simulink model "WindPlatform"  (Simulink 7.5)
settings: Solver=ode23s  StartTime=0.0  StopTime=700  RelTol=1e-3
InitFcn:
  | initialise
values from neighbouring files (symbols this model uses):
  B = 20/100    (= 0.2)    [initialise.m]    (also in windmodel.m)
  D = [6.5541e-04 0 0;0 7.1768e-04 -6.3413E-08;0 -2.1033E-08 -2.6495E-10]    [initialise.m]
  L = 30/100    (= 0.3)    [initialise.m]    (also in windmodel.m = 0.2)
  MA = [2.5 0 0 ... (first row only)    [initialise.m]
  MRB = [1.65 0 0 ... (first row only)    [initialise.m]
undefined symbols (not defined in the file or in its folder): effoceancurrent, magnitude, rotation, windmodel
libraries: simulink x3, marine_gnc x2, simulink_extras x2, instrumentlib x1, dspmtrx3 x1, aerolibutil x1
settings Model: Creator=Prasad  LastModifiedBy=Prasad
settings DebuggingCC: SolverPrmCheckMsg=none
settings SimEventsCC: propDiagAttribOutput=1  propDiagFcnCallOutput=1  propDiagStatOutput=0

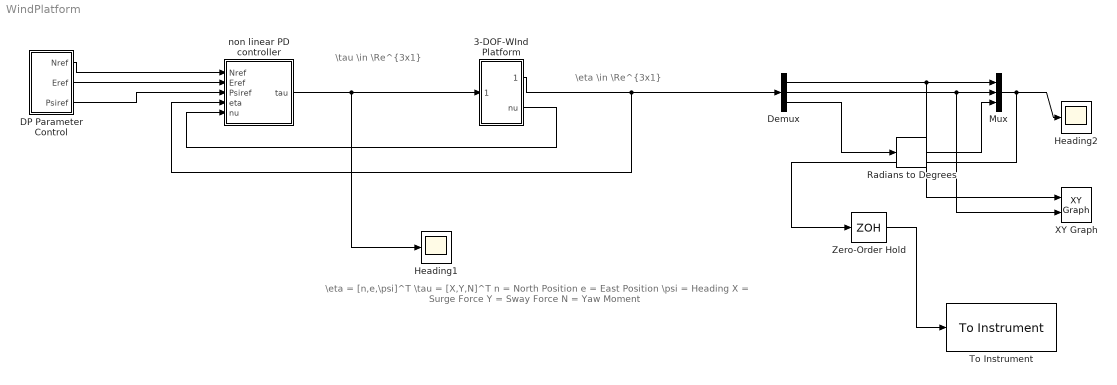
== system WindPlatform ==
  note: \tau \in \Re^{3x1}
  note: \eta \in \Re^{3x1}
  note: \eta = [n,e,\psi]^T
      | \tau = [X,Y,N]^T
      | n = North Position
      | e = East Position
      | \psi = Heading
      | X = Surge Force
      | Y = Sway Force
      | N = Yaw Moment
  3-DOF-WInd Platform : Subsystem
  DP Parameter Control : Subsystem  mask(Dynamic Position   ){geo=[10,20,100], k=[1 1 1], w=[0.05 0.05 0.05], zeta=[0.8 0.8 0.6]}
      mask prompts: geo "North-East-Heading[n,e,psi]"; k "Gain: [North East Heading]"; w "Time Constant: [North East Heading]"; zeta "Damping Factor: [North East Heading]"
      mask help: Set North-East(n,e) Positions of the vessel relative to the local geographical frame along with the heading angle relative to the north
      mask TabNameString: Basic,Advance,Advance,Advance
  Demux : Demux  Outputs=3
  Heading1 : Scope
      settings: TimeRange=700  YMin=-0.1  YMax=0.09
  Heading2 : Scope
      settings: TimeRange=700  YMin=-1  YMax=13
  Mux : Mux  Inputs=3
  Radians to Degrees : simulink_extras/Transformations/Radians to Degrees  SystemSampleTime=-1
  To Instrument : instrumentlib/To Instrument  sampleTime=-1  isWorkspaceObject=off  timeout=10  inputBufferSize=8192  protocol=UDP  serialPort=COM4  baudRate=9600  gpibVendor=Advantech  boardIndex=0  primaryAddress=1  secondaryAddress=0  visaVendor=Agilent  visaSerialPort=0  chassisIndex=0  logicalAddress=0  tcpRemoteHost='127.0.0.1'  tcpRemotePort=4500  udpRemoteHost='127.0.0.1'  udpRemotePort=9090  visaTCPBoardIndex=0  visaTCPRemoteHost='127.0.0.1'  usbBoardIndex=0  usbManufID=0  usbModelCode=0  usbSerialNumber=0  initAction=None  initCommand='DATA:SOURCE CH1'  initFunction=get  command='uw'  sendFormat=ASCII  asciiFormatting='%d'  precision=8-bit integer  byteOrder=Little endian
  XY Graph : simulink/Sinks/XY Graph  SystemSampleTime=-1  xmin=0  xmax=50  ymin=0  ymax=50  st=-1
  Zero-Order Hold : ZeroOrderHold
  non linear PD controller : Subsystem  mask(Non-Linear PD controller){kp=50*[1 0 0;1 0 0;0 0 2], kd=50}
      mask prompts: kp "Proportional Gain Kp"; kd "Derivative Gain Kd"
      mask help: Set proportional and derivative gains for the non-linear PD controller
  wires:
  Demux/1 -> Mux/1, XY Graph/1
  Demux/2 -> Mux/2, XY Graph/2
  Radians to Degrees/1 -> Mux/3
  DP Parameter Control/2(Eref) -> non linear PD controller/2(Eref)
  DP Parameter Control/1(Nref) -> non linear PD controller/1(Nref)
  Demux/3 -> Radians to Degrees/1
  3-DOF-WInd Platform/1(eta) -> non linear PD controller/4(eta), Demux/1
  3-DOF-WInd Platform/2(nu) -> non linear PD controller/5(nu)
  DP Parameter Control/3(Psiref) -> non linear PD controller/3(Psiref)
  non linear PD controller/1(tau) -> 3-DOF-WInd Platform/1(tau), Heading1/1
  Mux/1 -> Heading2/1, Zero-Order Hold/1
  Zero-Order Hold/1 -> To Instrument/1

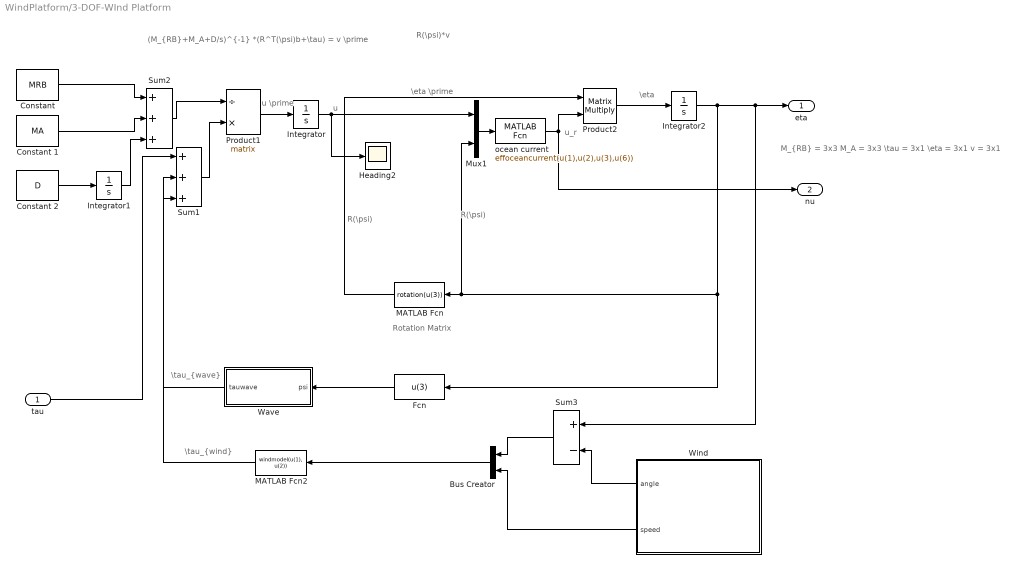
== system WindPlatform/3-DOF-WInd Platform ==
  note: (M_{RB}+M_A+D/s)^{-1} *(R^T(\psi)b+\tau) = v \prime
  note: \nu
  note: R(\psi)*v
  note: \eta
  note: M_{RB} = 3x3
      | M_A = 3x3
      | \tau = 3x1
      | \eta = 3x1
      | v = 3x1
  note: \nu \prime
  note: \eta \prime
  note: \tau_{wind}
  note: \nu_r
  note: \tau_{wave}
  note: R(\psi)
  note: R(\psi)
  note: Rotation Matrix
  tau : Inport  OutDataType=sfix(16)  OutScaling=2^0
  Bus Creator : BusCreator  Inputs=2
  "Constant " : Constant  Value=MRB  VectorParams1D=off  OutDataType=sfix(16)  OutScaling=2^0
  Constant 1 : Constant  Value=MA  VectorParams1D=off  OutDataType=sfix(16)  OutScaling=2^0
  Constant 2 : Constant  Value=D  VectorParams1D=off  OutDataType=sfix(16)  OutScaling=2^0
  Fcn : Fcn  Expr=u(3)
  Heading2 : Scope
      settings: TimeRange=700  YMin=-1.66533e-016  YMax=2.3  SaveName=ScopeData2
  Integrator : Integrator
  Integrator1 : Integrator
  Integrator2 : Integrator
  MATLAB Fcn : MATLABFcn  MATLABFcn=rotation(u(3))  OutputDimensions=[3 3]  Output1D=off
  MATLAB Fcn2 : MATLABFcn  MATLABFcn=windmodel(u(1), u(2))  OutputDimensions=[3 1]  Output1D=off
  Mux1 : Mux  Inputs=2
  Product1 : Product  Inputs=/*  Multiplication=Matrix(*)  OutDataType=sfix(16)  OutScaling=2^0  SaturateOnIntegerOverflow=on  OutDataTypeStr=Inherit: Same as first input
  Product2 : Product  Inputs=**  Multiplication=Matrix(*)  OutDataType=sfix(16)  OutScaling=2^0  OutDataTypeStr=Inherit: Same as first input
  Sum1 : Sum  Inputs=+++  OutDataType=sfix(16)  OutScaling=2^0  SaturateOnIntegerOverflow=on
  Sum2 : Sum  Inputs=+++  OutDataType=sfix(16)  OutScaling=2^0  SaturateOnIntegerOverflow=on
  Sum3 : Sum  Inputs=+-  OutDataType=sfix(16)  OutScaling=2^0  SaturateOnIntegerOverflow=on
  Wave : Subsystem
  Wind : Subsystem  AncestorBlock=marine_gnc/Environment/Wind/Wind  mask(Wind){page=2, Par_Wind_slowlyvar=on, Par_Wind_gust=on, Par_Wind_V=0.04, Par_Wind_angle=0, Par_Wind_spectrum_type=2, Par_Wind_z=0.01, Par_Wind_sample_time=0.01, Par_Wind_speed_T=100, Par_Wind_angle_T=10, Par_Wind_speed_noise_pow=0.001, Par_Wind_angle_noise_pow=0.001, Par_Wind_speed_rand_max=0.1, Par_Wind_angle_rand_max=pi/4, Par_Wind_speed_seed=1, Par_Wind_angle_seed=1, Par_Wind_phase_seed=1, Par_Wind_kappa_H=0.0026, Par_Wind_L=1800, Par_Wind_minfreq=1E-4, Par_Wind_maxfreq=0.1, Par_Wind_nfreq=10}
      mask prompts: Par_Wind_slowlyvar "Include slowly-varing wind velocity and direction"; Par_Wind_gust "Include wind gust"; Par_Wind_V "Mean wind velocity [m/s]"; Par_Wind_angle "Mean wind angle [rad]"; Par_Wind_spectrum_type "Wind gust spectrum type"; Par_Wind_z "Height over water surface [m (for NORSOK wind spectrum)]"; Par_Wind_sample_time "Wind sample time [s]"; Par_Wind_speed_T "Wind speed time constant [s]"; Par_Wind_angle_T "Wind angle time constant [s]"; Par_Wind_speed_noise_pow "Wind speed noise power"; Par_Wind_angle_noise_pow "Wind angle noise power"; Par_Wind_speed_rand_max "Wind speed saturation [m/s] (max random variation about mean)"; Par_Wind_angle_rand_max "Wind angle saturation [rad] (max random variation about mean)"; Par_Wind_speed_seed "Wind speed random seed"; Par_Wind_angle_seed "Wind angle random seed"; Par_Wind_phase_seed "Wind gust phase seed"; Par_Wind_kappa_H "Sea surface drag coefficient for Harris wind spectrum (0.0026)"; Par_Wind_L "Scaling length for Harris wind spectrum (1800)"; Par_Wind_minfreq "Minimum frequency in gust [Hz] (1E-4)"; Par_Wind_maxfreq "Maximum frequency in gust [Hz] (0.1)"; Par_Wind_nfreq "Number of frequency components"
      mask help:
      | Generates wind speed and direction based on the mean angle and mean wind speed at 10 meters height. The total velocity is composed of a slowly-varying mean superposed with gusts based on a chosen wind spectrum. The direction is slowly-varying based on a random process.
      |
      | The wind spectrum types are:
      |
      | 1) Harris         (based on measurements over land)
      | 2) NORSOK   (based on measurements from the North Sea)
      mask Help:
      | <b>Part of the Marine Systems Simulator: MSS</b><p>Generate wind speed and direction based on the mean angle and mean wind
      | speed at 10 meters height. The total velocity is composed of a slowly-varying
      | mean superposed with gusts based on a chosen wind spectrum. The direction is
      | slowly-varying based on a random process.<br>
      | <br>
      | The wind spectrum types are:<br>
      | <br>
      | 1) Harris (based on measurements over land)<br>
      | 2) NORSOK (based on measurements from the North Sea)</p>
      | <p>The wind gust from the Harris spectrum is uniform over the height, whereas
      | the wind gust from the NORSOK spectrum varies with the height.</p>
      | <p>The random variation of the mean speed and angle can be limited by two saturation
      | parameters, which define the maximum random deviation from the mean value.<p><b>Outputs:
      | </b> </p>
      | <p>angle: [rad] Wind angle in the n-frame<br>
      | speed: [m/s] Wind velocity in the n-frame<p>
      | <b>Copyright NTNU 2005</b></p>
      | <p><b>Author:</b> Oyvind N. Smogeli, 2005-05-03</p>
      mask StyleString: popup(1|2),checkbox,checkbox,edit,edit,popup(1|2),edit,edit,edit,edit,edit,edit,edit,edit,edit,edit,edit,edit,edit,edit,edit,edit
      mask CallbackString: MSS_mask_page(12);|||||||||||||||||||||
  ocean current : MATLABFcn  MATLABFcn=effoceancurrent(u(1),u(2),u(3),u(6))  OutputDimensions=[3 1]  Output1D=off
  eta : Outport  OutDataType=sfix(16)  OutScaling=2^0
  nu : Outport  Port=2  OutDataType=sfix(16)  OutScaling=2^0
  wires:
  Integrator/1 -> Mux1/1, Heading2/1
  Product2/1 -> Integrator2/1
  "Constant "/1 -> Sum2/1
  Constant 1/1 -> Sum2/2
  MATLAB Fcn/1 -> Product2/1
  Constant 2/1 -> Integrator1/1
  Product1/1 -> Integrator/1
  tau/1 -> Sum1/1
  Sum2/1 -> Product1/1
  Wind/1(angle) -> Sum3/2
  Sum3/1 -> Bus Creator/1
  Wind/2(speed) -> Bus Creator/2
  Bus Creator/1 -> MATLAB Fcn2/1
  Fcn/1 -> Wave/1(psi)
  Sum1/1 -> Product1/2
  Mux1/1 -> ocean current/1
  ocean current/1 -> nu/1, Product2/2
  Integrator2/1 -> MATLAB Fcn/1, Mux1/2, Fcn/1, eta/1, Sum3/1
  Wave/1(tauwave) -> Sum1/2
  Integrator1/1 -> Sum2/3
  MATLAB Fcn2/1 -> Sum1/3

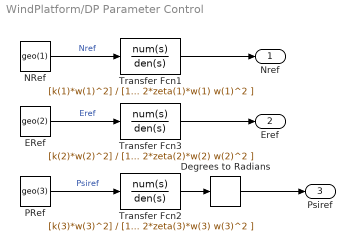
== system WindPlatform/DP Parameter Control ==
  Degrees to Radians : simulink_extras/Transformations/Degrees to Radians  SystemSampleTime=-1
  ERef : Constant  Value=geo(2)  OutDataType=fixdt(1, 16)  OutScaling=2^0
  NRef : Constant  Value=geo(1)  OutDataType=fixdt(1, 16)  OutScaling=2^0
  PRef : Constant  Value=geo(3)  OutDataType=fixdt(1, 16)  OutScaling=2^0
  Transfer Fcn1 : TransferFcn  Numerator=[k(1)*w(1)^2]  Denominator=[1 2*zeta(1)*w(1) w(1)^2 ]
  Transfer Fcn2 : TransferFcn  Numerator=[k(3)*w(3)^2]  Denominator="[1  2*zeta(3)*w(3) w(3)^2 ]"
  Transfer Fcn3 : TransferFcn  Numerator=[k(2)*w(2)^2]  Denominator="[1  2*zeta(2)*w(2) w(2)^2 ]"
  Nref : Outport
  Eref : Outport  Port=2
  Psiref : Outport  Port=3
  wires:
  Transfer Fcn2/1 -> Degrees to Radians/1
  NRef/1 -> Transfer Fcn1/1  "Nref"
  Transfer Fcn1/1 -> Nref/1
  ERef/1 -> Transfer Fcn3/1  "Eref"
  Transfer Fcn3/1 -> Eref/1
  PRef/1 -> Transfer Fcn2/1  "Psiref"
  Degrees to Radians/1 -> Psiref/1

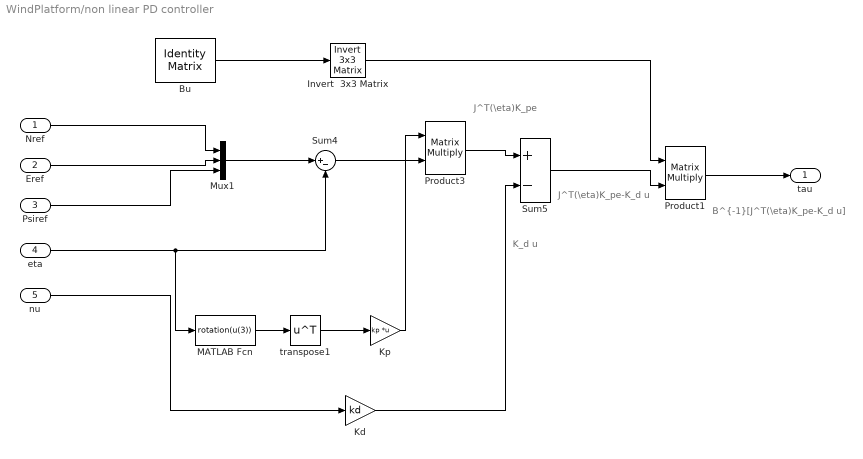
== system WindPlatform/non linear PD controller ==
  note: J^T(\eta)K_pe
  note: K_d\nu
  note: J^T(\eta)K_pe-K_d\nu
  note: B^{-1}[J^T(\eta)K_pe-K_d\nu]
  Nref : Inport
  Eref : Inport  Port=2
  Psiref : Inport  Port=3
  eta : Inport  Port=4
  nu : Inport  Port=5
  Bu : dspmtrx3/Identity Matrix  Inherit=off  N=3  Ts=1  dataType=double  isSigned=on  wordLen=16  udDataType=sfix(16)  fracBitsMode=Best precision  numFracBits=15
  Invert  3x3 Matrix : aerolibutil/Invert  3x3 Matrix  SystemSampleTime=-1
  Kd : Gain  Gain=kd  ParameterDataType=fixdt(1, 16)  ParameterScaling=2^0  OutDataType=fixdt(1, 16)  OutScaling=2^0
  Kp : Gain  Gain=kp  Multiplication=Matrix(K*u)  ParameterDataType=fixdt(1, 16)  ParameterScaling=2^0  OutDataType=fixdt(1, 16)  OutScaling=2^0
  MATLAB Fcn : MATLABFcn  MATLABFcn=rotation(u(3))  OutputDimensions=[3 3]  Output1D=off
  Mux1 : Mux  Inputs=3
  Product1 : Product  Inputs=**  Multiplication=Matrix(*)  OutDataType=sfix(16)  OutScaling=2^0  SaturateOnIntegerOverflow=on  OutDataTypeStr=Inherit: Same as first input
  Product3 : Product  Inputs=**  Multiplication=Matrix(*)  OutDataType=sfix(16)  OutScaling=2^0  SaturateOnIntegerOverflow=on  OutDataTypeStr=Inherit: Same as first input
  Sum4 : Sum  Inputs=|+-  OutDataType=fixdt(1, 16)  OutScaling=2^0
  Sum5 : Sum  Inputs=+-  OutDataType=sfix(16)  OutScaling=2^0  SaturateOnIntegerOverflow=on
  transpose1 : Math  Operator=transpose  OutDataType=sfix(16)  OutScaling=2^0  SaturateOnIntegerOverflow=on
  tau : Outport
  wires:
  Nref/1 -> Mux1/1
  Eref/1 -> Mux1/2
  Psiref/1 -> Mux1/3
  Product1/1 -> tau/1
  Mux1/1 -> Sum4/1
  eta/1 -> Sum4/2, MATLAB Fcn/1
  nu/1 -> Kd/1
  Bu/1 -> Invert  3x3 Matrix/1
  Product3/1 -> Sum5/1
  Kd/1 -> Sum5/2
  Invert  3x3 Matrix/1 -> Product1/1
  Sum5/1 -> Product1/2
  Sum4/1 -> Product3/2
  MATLAB Fcn/1 -> transpose1/1
  Kp/1 -> Product3/1
  transpose1/1 -> Kp/1

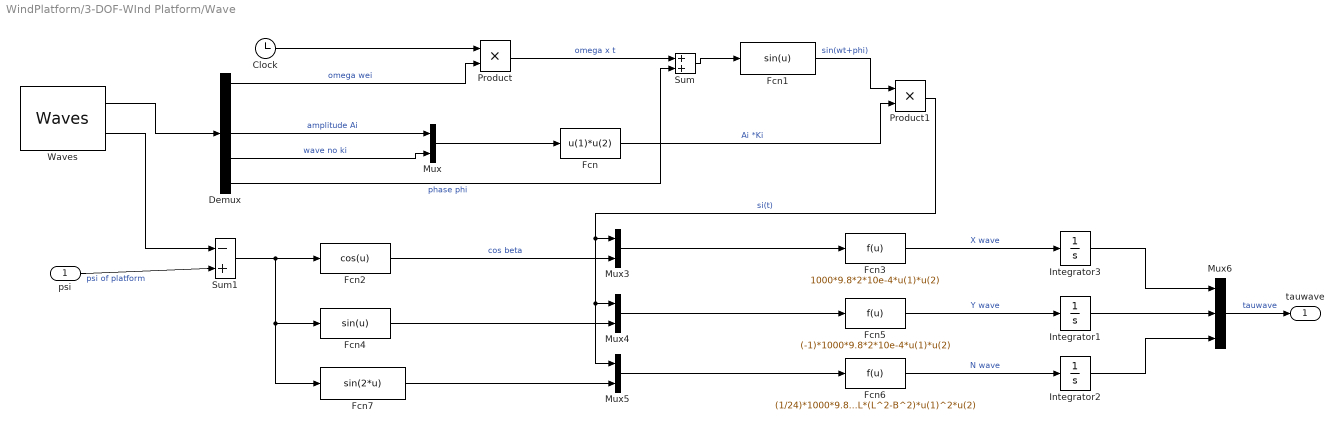
== system WindPlatform/3-DOF-WInd Platform/Wave ==
  psi : Inport  OutDataType=fixdt(1, 16)  OutScaling=2^0
  Clock : Clock
      settings: Decimation=10
  Demux : Demux  Outputs=5
  Fcn : Fcn  Expr=u(1)*u(2)
  Fcn1 : Fcn  Expr=sin(u)
  Fcn2 : Fcn  Expr=cos(u)
  Fcn3 : Fcn  Expr=1000*9.8*2*10e-4*u(1)*u(2)
  Fcn4 : Fcn  Expr=sin(u)
  Fcn5 : Fcn  Expr=(-1)*1000*9.8*2*10e-4*u(1)*u(2)
  Fcn6 : Fcn  Expr=(1/24)*1000*9.8*B*L*(L^2-B^2)*u(1)^2*u(2)
  Fcn7 : Fcn  Expr=sin(2*u)
  Integrator1 : Integrator
  Integrator2 : Integrator
  Integrator3 : Integrator
  Mux{,3..5} (4 alike) : Mux  Inputs=2
  Mux6 : Mux  Inputs=3
  Product : Product  OutDataType=fixdt(1, 16)  OutScaling=2^0  RndMeth=Zero
  Product1 : Product  OutDataType=fixdt(1, 16)  OutScaling=2^0  RndMeth=Zero
  Sum : Sum  Inputs=+|+  OutDataType=fixdt(1, 16)  OutScaling=2^0
  Sum1 : Sum  Inputs=-|+  OutDataType=fixdt(1, 16)  OutScaling=2^0
  Waves : marine_gnc/Environment/Waves/Waves  SystemSampleTime=-1  spectrum_type=ITTC  disp_flag=on  plot_spectrum=off  plot_realization=off  hs=0.15  omega_peak=0.984  psi_mean=0  gamma=-1  spread=2  depth=inf  nfreq=20  ndir=10  energylim=0.005  freq_cutoff=3  dir_cutoff=0  rand_seed=123  rand_freq=on  rand_dir=on  Zeta_a=0  Omega=0  Phase=0  Wavenum=0  Psi=0
  tauwave : Outport  OutDataType=fixdt(1, 16)  OutScaling=2^0
  wires:
  Waves/1 -> Demux/1
  Demux/3 -> Mux/1  "amplitude Ai"
  Demux/4 -> Mux/2  "wave no ki"
  Mux/1 -> Fcn/1
  Clock/1 -> Product/1
  Demux/1 -> Product/2  "omega wei"
  Fcn1/1 -> Product1/1  "sin(wt+phi)"
  Sum1/1 -> Fcn2/1, Fcn4/1, Fcn7/1
  Mux3/1 -> Fcn3/1
  Mux4/1 -> Fcn5/1
  Mux5/1 -> Fcn6/1
  Product/1 -> Sum/1  "omega x t"
  Sum/1 -> Fcn1/1
  Demux/5 -> Sum/2  "phase phi"
  psi/1 -> Sum1/2  "psi of platform"
  Waves/2 -> Sum1/1
  Fcn3/1 -> Integrator3/1  "X wave"
  Fcn6/1 -> Integrator2/1  "N wave"
  Fcn/1 -> Product1/2  "Ai *Ki"
  Product1/1 -> Mux3/1, Mux4/1, Mux5/1  "si(t)"
  Fcn2/1 -> Mux3/2  "cos beta"
  Fcn4/1 -> Mux4/2
  Fcn7/1 -> Mux5/2
  Fcn5/1 -> Integrator1/1  "Y wave"
  Integrator3/1 -> Mux6/1
  Integrator1/1 -> Mux6/2
  Integrator2/1 -> Mux6/3
  Mux6/1 -> tauwave/1  "tauwave"

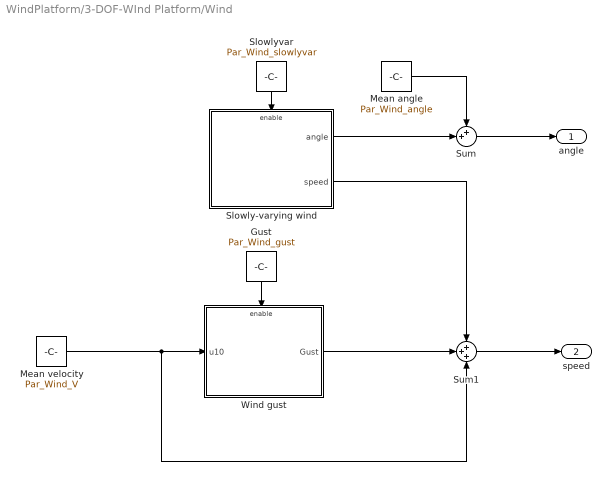
== system WindPlatform/3-DOF-WInd Platform/Wind ==
  Gust : Constant  Value=Par_Wind_gust  OutDataType=sfix(16)  OutScaling=2^0
  Mean angle : Constant  Value=Par_Wind_angle  OutDataType=sfix(16)  OutScaling=2^0
  Mean velocity : Constant  Value=Par_Wind_V  OutDataType=sfix(16)  OutScaling=2^0
  Slowly-varying wind : Subsystem  mask(Slowly-varying wind){Par_Wind_sample_time=Par_Wind_sample_time, Par_Wind_speed_T=Par_Wind_speed_T, Par_Wind_angle_T=Par_Wind_angle_T, Par_Wind_speed_noise_pow=Par_Wind_speed_noise_pow, Par_Wind_angle_noise_pow=Par_Wind_angle_noise_pow, Par_Wind_speed_rand_max=Par_Wind_speed_rand_max, Par_Wind_angle_rand_max=Par_Wind_angle_rand_max, Par_Wind_speed_seed=Par_Wind_speed_seed, Par_Wind_angle_seed=Par_Wind_angle_seed}
      mask prompts: Par_Wind_sample_time "Wind sample time [s]"; Par_Wind_speed_T "Wind speed time constant [s]"; Par_Wind_angle_T "Wind angle time constant [s]"; Par_Wind_speed_noise_pow "Wind speed noise power"; Par_Wind_angle_noise_pow "Wind angle noise power"; Par_Wind_speed_rand_max "Wind speed saturation [m/s] (max random variation about mean)"; Par_Wind_angle_rand_max "Wind angle saturation [rad] (max random variation about mean)"; Par_Wind_speed_seed "Wind speed random seed"; Par_Wind_angle_seed "Wind angle random seed"
      mask help:
      | Generate slowly varying wind speed and direction based on random processes.
      |
      | stochastic = 0  gives constant mean wind speed and direction
      | stochastic = 1  gives stochastic mean wind speed and direction
      mask Help:
      | Generate slowly varying wind speed and direction based on random processes.<br>
      | <br>
      | stochastic = 0 gives constant mean wind direction and speed,<br>
      | stochastic = 1 gives stochastic mean wind direction and speed<br>
      | <br>
      | <p>The randomness of the mean speed and angle can be limited by two saturation
      | parameters, which define the maximum random deviation from the mean value.<br>
  Slowlyvar : Constant  Value=Par_Wind_slowlyvar  OutDataType=sfix(16)  OutScaling=2^0
  Sum : Sum  Inputs=++|  OutDataType=sfix(16)  OutScaling=2^0  SaturateOnIntegerOverflow=on
  Sum1 : Sum  Inputs=+++  OutDataType=sfix(16)  OutScaling=2^0  SaturateOnIntegerOverflow=on
  Wind gust : Subsystem  mask(Wind gust){Par_Wind_spectrum_type=Par_Wind_spectrum_type, Par_Wind_phase_seed=Par_Wind_phase_seed, Par_Wind_kappa_H=Par_Wind_kappa_H, Par_Wind_L=Par_Wind_L, Par_Wind_z=Par_Wind_z, Par_Wind_minfreq=Par_Wind_minfreq, Par_Wind_maxfreq=Par_Wind_maxfreq, Par_Wind_nfreq=Par_Wind_nfreq}
      mask prompts: Par_Wind_spectrum_type "Spectrum type"; Par_Wind_phase_seed "Wind gust phase seed"; Par_Wind_kappa_H "Sea surface drag coefficient for Harris wind spectrum (0.0026)"; Par_Wind_L "Scaling length for Harris wind spectrum (1800)"; Par_Wind_z "Height over water surface, for NORSOK spectrum"; Par_Wind_minfreq "Minimum frequency in gust [Hz] (1E-4)"; Par_Wind_maxfreq "Maximum frequency in gust [Hz] (0.1)"; Par_Wind_nfreq "Number of frequency components"
      mask help:
      | Calculate the wind gust according to one of two gust spectra:
      |
      | 1) Harris (based on measurements over land)
      | 2) NORSOK (based on measurements from the North Sea)
      |
      | The gust from the Harris spectrum is not influenced by the heigth over the sea surface, whereas the gust from the NORSOK spectrum is.
  angle : Outport  OutDataType=sfix(16)  OutScaling=2^0
  speed : Outport  Port=2  OutDataType=sfix(16)  OutScaling=2^0
  wires:
  Sum1/1 -> speed/1
  Slowly-varying wind/2(speed) -> Sum1/1
  Wind gust/1(Gust) -> Sum1/2
  Sum/1 -> angle/1
  Mean angle/1 -> Sum/1
  Mean velocity/1 -> Sum1/3, Wind gust/1(u10)
  Slowly-varying wind/1(angle) -> Sum/2
  Slowlyvar/1 -> Slowly-varying wind/Enable
  Gust/1 -> Wind gust/Enable

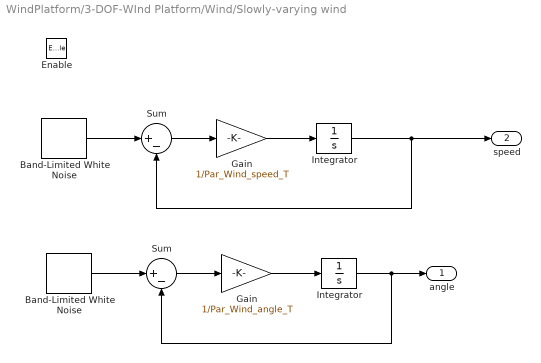
== system WindPlatform/3-DOF-WInd Platform/Wind/Slowly-varying wind ==
  Enable : EnablePort
  Band-Limited White Noise : simulink/Sources/Band-Limited White Noise  SystemSampleTime=-1  Cov=Par_Wind_speed_noise_pow  Ts=Par_Wind_sample_time  seed=Par_Wind_speed_seed
  "Band-Limited White Noise " : simulink/Sources/Band-Limited White Noise  SystemSampleTime=-1  Cov=Par_Wind_angle_noise_pow  Ts=Par_Wind_sample_time  seed=Par_Wind_angle_seed
  Gain : Gain  Gain=1/Par_Wind_speed_T  ParameterDataType=sfix(16)  ParameterScaling=2^0  OutDataType=sfix(16)  OutScaling=2^0  SaturateOnIntegerOverflow=on  OutDataTypeStr=Inherit: Same as input  ParamDataTypeStr=Inherit: Same as input
  "Gain " : Gain  Gain=1/Par_Wind_angle_T  ParameterDataType=sfix(16)  ParameterScaling=2^0  OutDataType=sfix(16)  OutScaling=2^0  SaturateOnIntegerOverflow=on  OutDataTypeStr=Inherit: Same as input  ParamDataTypeStr=Inherit: Same as input
  Integrator : Integrator  LimitOutput=on  UpperSaturationLimit=Par_Wind_speed_rand_max  LowerSaturationLimit=-Par_Wind_speed_rand_max
  "Integrator " : Integrator  LimitOutput=on  UpperSaturationLimit=Par_Wind_angle_rand_max  LowerSaturationLimit=-Par_Wind_angle_rand_max
  Sum : Sum  Inputs=|+-  OutDataType=sfix(16)  OutScaling=2^0  SaturateOnIntegerOverflow=on  InputSameDT=on  OutDataTypeStr=Inherit: Same as first input
  "Sum       " : Sum  Inputs=|+-  OutDataType=sfix(16)  OutScaling=2^0  SaturateOnIntegerOverflow=on  InputSameDT=on  OutDataTypeStr=Inherit: Same as first input
  angle : Outport  OutDataType=sfix(16)  OutScaling=2^0  InitialOutput=0
  speed : Outport  Port=2  OutDataType=sfix(16)  OutScaling=2^0  InitialOutput=0
  wires:
  "Gain "/1 -> "Integrator "/1
  "Sum       "/1 -> "Gain "/1
  "Integrator "/1 -> angle/1, "Sum       "/2
  "Band-Limited White Noise "/1 -> "Sum       "/1
  Gain/1 -> Integrator/1
  Sum/1 -> Gain/1
  Integrator/1 -> speed/1, Sum/2
  Band-Limited White Noise/1 -> Sum/1

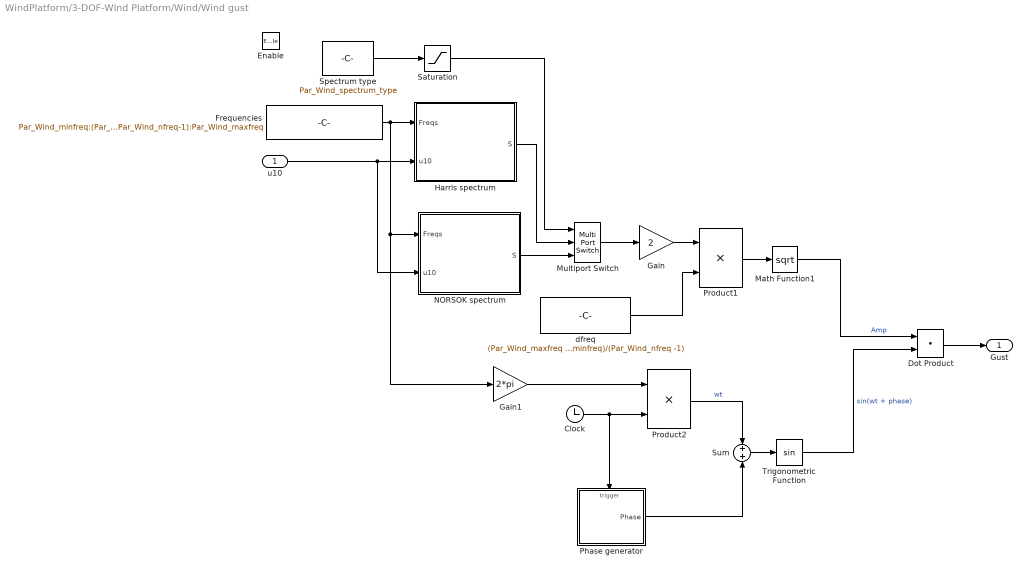
== system WindPlatform/3-DOF-WInd Platform/Wind/Wind gust ==
  u10 : Inport  OutDataType=sfix(16)  OutScaling=2^0
  Enable : EnablePort
  Clock : Clock
      settings: Decimation=10
  Dot Product : DotProduct  OutDataType=sfix(16)  OutScaling=2^-10  InputSameDT=on  OutDataTypeStr=Inherit: Inherit via internal rule
  Frequencies : Constant  Value=Par_Wind_minfreq:(Par_Wind_maxfreq - Par_Wind_minfreq)/(Par_Wind_nfreq-1):Par_Wind_maxfreq  OutDataType=sfix(16)  OutScaling=2^0
  Gain : Gain  Gain=2  ParameterDataType=sfix(16)  ParameterScaling=2^0  OutDataType=sfix(16)  OutScaling=2^0  SaturateOnIntegerOverflow=on  OutDataTypeStr=Inherit: Same as input  ParamDataTypeStr=Inherit: Same as input
  Gain1 : Gain  Gain=2*pi  ParameterDataType=sfix(16)  ParameterScaling=2^0  OutDataType=sfix(16)  OutScaling=2^0  SaturateOnIntegerOverflow=on  OutDataTypeStr=Inherit: Same as input  ParamDataTypeStr=Inherit: Same as input
  Harris spectrum : Subsystem
  Math Function1 : Math  Operator=sqrt  OutDataType=sfix(16)  OutScaling=2^0  SaturateOnIntegerOverflow=on
  Multiport Switch : MultiPortSwitch  Inputs=2  zeroidx=off  RndMeth=Nearest  SaturateOnIntegerOverflow=on
  NORSOK spectrum : Subsystem
  Phase generator : Subsystem
  Product1 : Product  OutDataType=sfix(16)  OutScaling=2^0  SaturateOnIntegerOverflow=on  OutDataTypeStr=Inherit: Same as first input
  Product2 : Product  OutDataType=sfix(16)  OutScaling=2^0  SaturateOnIntegerOverflow=on  OutDataTypeStr=Inherit: Same as first input
  Saturation : Saturate  UpperLimit=2  LowerLimit=1
  Spectrum type : Constant  Value=Par_Wind_spectrum_type  OutDataType=sfix(16)  OutScaling=2^0
  Sum : Sum  OutDataType=sfix(16)  OutScaling=2^0  SaturateOnIntegerOverflow=on
  Trigonometric Function : Trigonometry
  dfreq : Constant  Value=(Par_Wind_maxfreq - Par_Wind_minfreq)/(Par_Wind_nfreq -1)  OutDataType=sfix(16)  OutScaling=2^0
  Gust : Outport  OutDataType=sfix(16)  OutScaling=2^0  InitialOutput=0
  wires:
  Dot Product/1 -> Gust/1
  Trigonometric Function/1 -> Dot Product/2  "sin(wt + phase)"
  Math Function1/1 -> Dot Product/1  "Amp"
  Sum/1 -> Trigonometric Function/1
  Phase generator/1(Phase) -> Sum/2
  Product2/1 -> Sum/1  "wt"
  Clock/1 -> Phase generator/Trigger, Product2/2
  Gain1/1 -> Product2/1
  NORSOK spectrum/1(S) -> Multiport Switch/3
  Harris spectrum/1(S) -> Multiport Switch/2
  Spectrum type/1 -> Saturation/1
  Multiport Switch/1 -> Gain/1
  Product1/1 -> Math Function1/1
  dfreq/1 -> Product1/2
  Gain/1 -> Product1/1
  u10/1 -> Harris spectrum/2(u10), NORSOK spectrum/2(u10)
  Frequencies/1 -> Gain1/1, NORSOK spectrum/1(Freqs), Harris spectrum/1(Freqs)
  Saturation/1 -> Multiport Switch/1

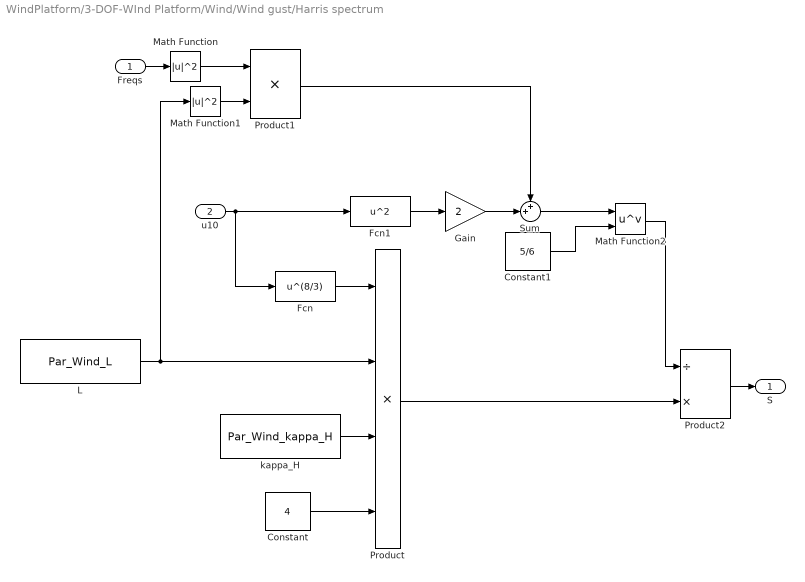
== system WindPlatform/3-DOF-WInd Platform/Wind/Wind gust/Harris spectrum ==
  Freqs : Inport  OutDataType=sfix(16)  OutScaling=2^0
  u10 : Inport  Port=2  OutDataType=sfix(16)  OutScaling=2^0
  Constant : Constant  Value=4  OutDataType=sfix(16)  OutScaling=2^0
  Constant1 : Constant  Value=5/6  OutDataType=sfix(16)  OutScaling=2^0
  Fcn : Fcn  Expr=u^(8/3)
  Fcn1 : Fcn  Expr=u^2
  Gain : Gain  Gain=2  ParameterDataType=sfix(16)  ParameterScaling=2^0  OutDataType=sfix(16)  OutScaling=2^0  SaturateOnIntegerOverflow=on  OutDataTypeStr=Inherit: Same as input  ParamDataTypeStr=Inherit: Same as input
  L : Constant  Value=Par_Wind_L  OutDataType=sfix(16)  OutScaling=2^0
  Math Function : Math  Operator=magnitude^2  OutDataType=sfix(16)  OutScaling=2^0  SaturateOnIntegerOverflow=on
  Math Function1 : Math  Operator=magnitude^2  OutDataType=sfix(16)  OutScaling=2^0  SaturateOnIntegerOverflow=on
  Math Function2 : Math  Operator=pow  OutDataType=sfix(16)  OutScaling=2^0  SaturateOnIntegerOverflow=on
  Product : Product  Inputs=4  OutDataType=sfix(16)  OutScaling=2^0  SaturateOnIntegerOverflow=on  OutDataTypeStr=Inherit: Same as first input
  Product1 : Product  OutDataType=sfix(16)  OutScaling=2^0  SaturateOnIntegerOverflow=on  OutDataTypeStr=Inherit: Same as first input
  Product2 : Product  Inputs=/*  OutDataType=sfix(16)  OutScaling=2^0  SaturateOnIntegerOverflow=on  OutDataTypeStr=Inherit: Same as first input
  Sum : Sum  Inputs=++|  OutDataType=sfix(16)  OutScaling=2^0  SaturateOnIntegerOverflow=on
  kappa_H : Constant  Value=Par_Wind_kappa_H  OutDataType=sfix(16)  OutScaling=2^0
  S : Outport  OutDataType=sfix(16)  OutScaling=2^0
  wires:
  Product2/1 -> S/1
  Freqs/1 -> Math Function/1
  Product/1 -> Product2/2
  Math Function2/1 -> Product2/1
  Constant1/1 -> Math Function2/2
  Sum/1 -> Math Function2/1
  Product1/1 -> Sum/1
  Math Function1/1 -> Product1/2
  Math Function/1 -> Product1/1
  L/1 -> Math Function1/1, Product/2
  Constant/1 -> Product/4
  Gain/1 -> Sum/2
  Fcn1/1 -> Gain/1
  u10/1 -> Fcn/1, Fcn1/1
  Fcn/1 -> Product/1
  kappa_H/1 -> Product/3

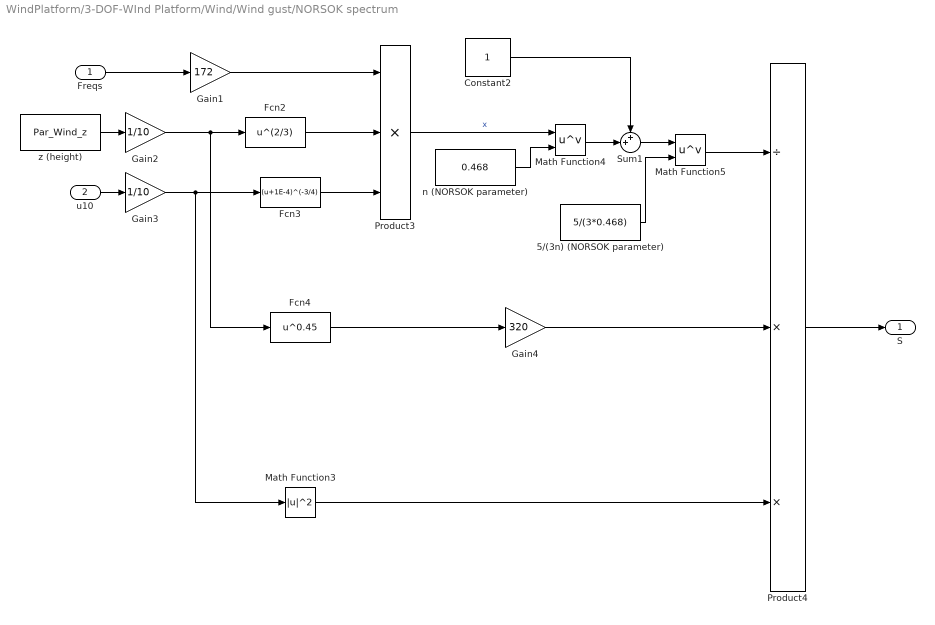
== system WindPlatform/3-DOF-WInd Platform/Wind/Wind gust/NORSOK spectrum ==
  Freqs : Inport  OutDataType=sfix(16)  OutScaling=2^0
  u10 : Inport  Port=2  OutDataType=sfix(16)  OutScaling=2^0
  5/(3n) (NORSOK parameter) : Constant  Value=5/(3*0.468)  OutDataType=sfix(16)  OutScaling=2^0
  Constant2 : Constant  OutDataType=sfix(16)  OutScaling=2^0
  Fcn2 : Fcn  Expr=u^(2/3)
  Fcn3 : Fcn  Expr=(u+1E-4)^(-3/4)
  Fcn4 : Fcn  Expr=u^0.45
  Gain1 : Gain  Gain=172  ParameterDataType=sfix(16)  ParameterScaling=2^0  OutDataType=sfix(16)  OutScaling=2^0  SaturateOnIntegerOverflow=on  OutDataTypeStr=Inherit: Same as input  ParamDataTypeStr=Inherit: Same as input
  Gain2 : Gain  Gain=1/10  ParameterDataType=sfix(16)  ParameterScaling=2^0  OutDataType=sfix(16)  OutScaling=2^0  SaturateOnIntegerOverflow=on  OutDataTypeStr=Inherit: Same as input  ParamDataTypeStr=Inherit: Same as input
  Gain3 : Gain  Gain=1/10  ParameterDataType=sfix(16)  ParameterScaling=2^0  OutDataType=sfix(16)  OutScaling=2^0  SaturateOnIntegerOverflow=on  OutDataTypeStr=Inherit: Same as input  ParamDataTypeStr=Inherit: Same as input
  Gain4 : Gain  Gain=320  ParameterDataType=sfix(16)  ParameterScaling=2^0  OutDataType=sfix(16)  OutScaling=2^0  SaturateOnIntegerOverflow=on  OutDataTypeStr=Inherit: Same as input  ParamDataTypeStr=Inherit: Same as input
  Math Function3 : Math  Operator=magnitude^2  OutDataType=sfix(16)  OutScaling=2^0  SaturateOnIntegerOverflow=on
  Math Function4 : Math  Operator=pow  OutDataType=sfix(16)  OutScaling=2^0  SaturateOnIntegerOverflow=on
  Math Function5 : Math  Operator=pow  OutDataType=sfix(16)  OutScaling=2^0  SaturateOnIntegerOverflow=on
  Product3 : Product  Inputs=3  OutDataType=sfix(16)  OutScaling=2^0  SaturateOnIntegerOverflow=on  OutDataTypeStr=Inherit: Same as first input
  Product4 : Product  Inputs=/**  OutDataType=sfix(16)  OutScaling=2^0  SaturateOnIntegerOverflow=on  OutDataTypeStr=Inherit: Same as first input
  Sum1 : Sum  Inputs=++|  OutDataType=sfix(16)  OutScaling=2^0  SaturateOnIntegerOverflow=on
  n (NORSOK parameter) : Constant  Value=0.468  OutDataType=sfix(16)  OutScaling=2^0
  z (height) : Constant  Value=Par_Wind_z  OutDataType=sfix(16)  OutScaling=2^0
  S : Outport  OutDataType=sfix(16)  OutScaling=2^0
  wires:
  5/(3n) (NORSOK parameter)/1 -> Math Function5/2
  Product4/1 -> S/1
  Gain4/1 -> Product4/2
  Math Function3/1 -> Product4/3
  Fcn4/1 -> Gain4/1
  Math Function5/1 -> Product4/1
  Sum1/1 -> Math Function5/1
  Constant2/1 -> Sum1/1
  Math Function4/1 -> Sum1/2
  n (NORSOK parameter)/1 -> Math Function4/2
  Product3/1 -> Math Function4/1  "x"
  Fcn3/1 -> Product3/3
  Gain3/1 -> Math Function3/1, Fcn3/1
  u10/1 -> Gain3/1
  Fcn2/1 -> Product3/2
  Gain2/1 -> Fcn4/1, Fcn2/1
  z (height)/1 -> Gain2/1
  Gain1/1 -> Product3/1
  Freqs/1 -> Gain1/1

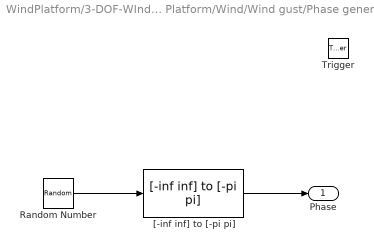
== system WindPlatform/3-DOF-WInd Platform/Wind/Wind gust/Phase generator ==
  Trigger : TriggerPort
  Random Number : RandomNumber  Variance=3  Seed=Par_Wind_phase_seed*[1:Par_Wind_nfreq]
  "[-inf inf] to [-pi pi]" : marine_gnc/Utilities/Math Operations/[-inf inf] to [-pi pi]  SystemSampleTime=-1
  Phase : Outport  OutDataType=sfix(16)  OutScaling=2^0
  wires:
  Random Number/1 -> "[-inf inf] to [-pi pi]"/1
  "[-inf inf] to [-pi pi]"/1 -> Phase/1
